simulink model "SolarPowered_chembattery2021b"  (R2021b)
settings: Solver=ode1  StartTime=0.0  StopTime=8760  FixedStep=1  RelTol=1e-3
undefined symbols (not defined in the file or in its folder): DiscIntNeverNeededParam
settings Model: Creator=alber  LastModifiedBy=alber
settings DebuggingCC: UnconnectedInputMsg=none  UnconnectedOutputMsg=none  UnconnectedLineMsg=none
settings ModelReferenceCC: EnableRefExpFcnMdlSchedulingChecks=off
settings RTWCC: DLArmComputeVersion=20.02.1

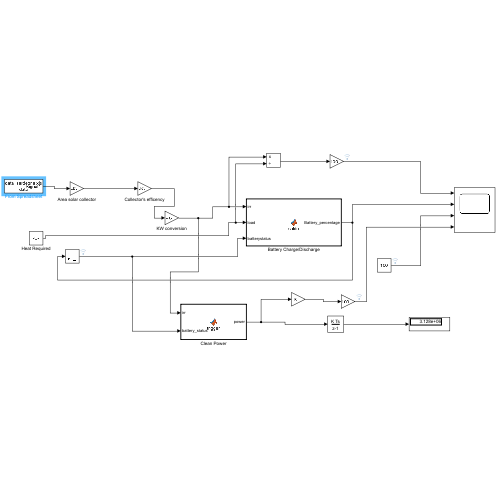
[thumbnail: Simulink's stored preview of the top-level diagram]
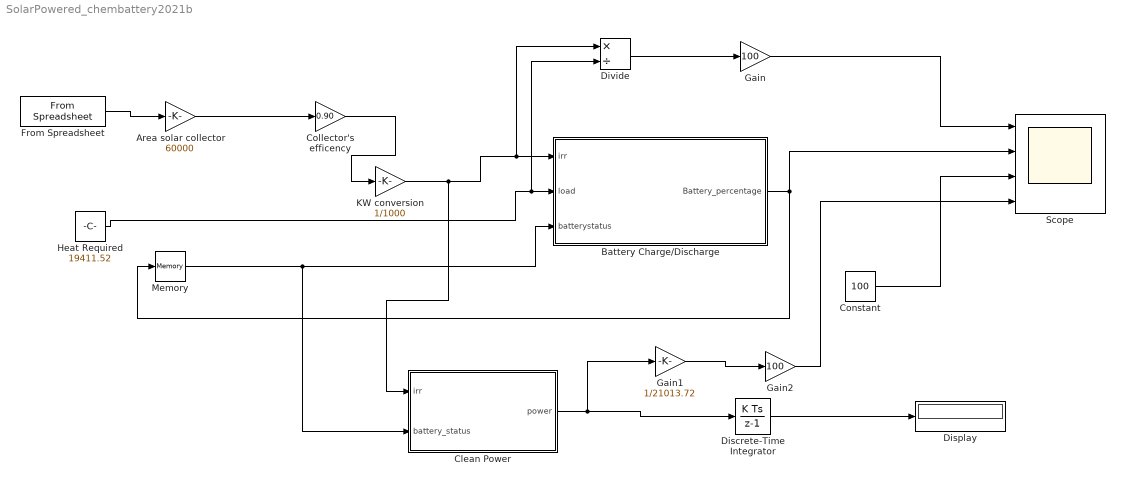
== system SolarPowered_chembattery2021b ==
  Area solar collector : Gain  Gain=60000
  Battery Charge/Discharge : MATLAB Function  TreatAsAtomicUnit=on
  Clean Power : MATLAB Function  TreatAsAtomicUnit=on
  Collector's efficency : Gain  Gain=0.90
  Constant : Constant  Value=100
  Discrete-Time Integrator : DiscreteIntegrator  SampleTime=-1  ICPrevOutput=DiscIntNeverNeededParam  ICPrevScaledInput=DiscIntNeverNeededParam
  Display : Display
  Divide : Product  Inputs=*/
  From Spreadsheet : FromSpreadsheet  FileName=data_sardegna.xls  SheetName=data  Range=A2:B8784
  Gain : Gain  Gain=100
  Gain1 : Gain  Gain=1/21013.72
  Gain2 : Gain  Gain=100
  Heat Required : Constant  Value=19411.52
  KW conversion : Gain  Gain=1/1000
  Memory : Memory  InitialCondition=100
  Scope : Scope  NumInputPorts=4
  wires:
  From Spreadsheet/1 -> Area solar collector/1
  Area solar collector/1 -> Collector's efficency/1
  Collector's efficency/1 -> KW conversion/1
  KW conversion/1 -> Clean Power/1(irr), Divide/1, Battery Charge/Discharge/1(irr)
  Heat Required/1 -> Divide/2, Battery Charge/Discharge/2(load)
  Memory/1 -> Clean Power/2(battery_status), Battery Charge/Discharge/3(batterystatus)
  Battery Charge/Discharge/1(Battery_percentage) -> Memory/1, Scope/2
  Divide/1 -> Gain/1
  Gain/1 -> Scope/1
  Constant/1 -> Scope/3
  Clean Power/1(power) -> Gain1/1, Discrete-Time Integrator/1
  Discrete-Time Integrator/1 -> Display/1
  Gain1/1 -> Gain2/1
  Gain2/1 -> Scope/4

== matlab function SolarPowered_chembattery2021b/Battery Charge//Discharge ==
  data: irr input; Battery_percentage output; load input; batterystatus input
function Battery_percentage = saldo(irr,load,batterystatus)
Battery_percentage = 0;
Delta = irr-load;
if Delta < 0
    if batterystatus > 0
        Battery_percentage = batterystatus-1;
        if Battery_percentage < 0
            Battery_percentage = 0;
        end
        return
    elseif batterystatus <= 0
        Battery_percentage = 0;
        return
    end
end
if Delta >=0
    if batterystatus ~= 100
        charge = (irr*0.025274)/49061.21 *100;
        Battery_percentage = batterystatus + charge;
        if Battery_percentage > 100
            Battery_percentage = 100;
        end
        return
    elseif batterystatus == 100
        Battery_percentage = 100;
        return
    end
end

== matlab function SolarPowered_chembattery2021b/Clean Power ==
  data: irr input; power output; battery_status input
function power = trigger(irr,battery_status)
Steam_trigger = 21013.72;
power = 0;
if battery_status == 100
    if irr < Steam_trigger
        power = 0;
        return
    else
        power = irr;
    end
end
end
